simulink model "gm_uz_pmsm_model_6LUT_pd_vnl"  (R2023b)
settings: Solver=FixedStepAuto  StartTime=0.0  StopTime=0.05  RelTol=1e-3
PreLoadFcn:
  | uz_pmsm_model_init_parameter
PostLoadFcn:
  | % Import the data from Excel for a lookup table
  | FluxMapData = readtable('C:\Users\Philipp\ultrazohm\ultrazohm_sw\ip_cores\uz_pmsm_model\FluxMapData_2023-05-26_13-07-57.csv');
  | % Row indices for lookup table
  | d_current_in_d_axis = FluxMapData(8:27,1:end);
  | % Column indices for lookup table
  | q_current_in_d_axis = FluxMapData(29:48,1:end);
  | % Output values for lookup table
  | d_Flux_d_axis = FluxMapData(50:69,1:end);
undefined symbols (not defined in the file or in its folder): ad1, ad2, ad3, ad4, ad5, ad6, aq1, aq2, aq3, aq4, aq5, aq6, d_current_d_Flux, d_current_q_Flux, entkopplung_dynamic, entkopplung_linear, entkopplung_static, Fid1_Giq1, Fid2_Giq2, Flux_d, Flux_q, friction_coefficient, inertia, Ki_Bo_d, Ki_Bo_q, Kp_Bo_d, Kp_Bo_q, L_d, L_q, Ldq, parameter_nachfuerung, polepair, praediktion_entkopplung_nonlinear, psi_pm, q_current_d_Flux, q_current_q_Flux, R_1, simulate_mechanical, simulate_nonlinear_modell, simulate_open_loop, static_friction_torque, tau_sum, ts, ts_regler
libraries: hdlmdlgenlib x19, simulink x2, slpidlib x2
(part 3 of 4)

== system gm_uz_pmsm_model_6LUT_pd_vnl/Current_Controller/Psi_d_q ==
  I_d_set : Inport
  I_d : Inport  Port=2
  I_q_set : Inport  Port=3
  I_q : Inport  Port=4
  Flux_d Lookup Table : Lookup_n-D  BreakpointsForDimension1=d_current_d_Flux  BreakpointsForDimension2=q_current_d_Flux  BreakpointsForDimension3=[5, 7]  Table=Flux_d  InternalRulePriority=Speed  RndMeth=Simplest
      settings: InputPortMap=u0,u1
  Flux_d Lookup Table1 : Lookup_n-D  BreakpointsForDimension1=d_current_d_Flux  BreakpointsForDimension2=q_current_d_Flux  BreakpointsForDimension3=[5, 7]  Table=Flux_d  InternalRulePriority=Speed  RndMeth=Simplest
      settings: InputPortMap=u0,u1
  Flux_q Lookup Table1 : Lookup_n-D  BreakpointsForDimension1=d_current_q_Flux  BreakpointsForDimension2=q_current_q_Flux  BreakpointsForDimension3=[5, 7]  Table=Flux_q  InternalRulePriority=Speed  RndMeth=Simplest
      settings: InputPortMap=u0,u1
  Flux_q Lookup Table2 : Lookup_n-D  BreakpointsForDimension1=d_current_q_Flux  BreakpointsForDimension2=q_current_q_Flux  BreakpointsForDimension3=[5, 7]  Table=Flux_q  InternalRulePriority=Speed  RndMeth=Simplest
      settings: InputPortMap=u0,u1
  Ldq Lookup Table : Lookup_n-D  BreakpointsForDimension1=d_current_q_Flux  BreakpointsForDimension2=q_current_q_Flux  BreakpointsForDimension3=[5, 7]  Table=Ldq  ExtrapMethod=Clip  UseLastTableValue=on  InternalRulePriority=Speed  OutDataTypeStr=Inherit: Inherit from 'Table data'  RndMeth=Simplest
      settings: InputPortMap=u0,u1
  Lqd Lookup Table1 : Lookup_n-D  BreakpointsForDimension1=d_current_q_Flux  BreakpointsForDimension2=q_current_q_Flux  BreakpointsForDimension3=[5, 7]  Table=Ldq  ExtrapMethod=Clip  UseLastTableValue=on  InternalRulePriority=Speed  OutDataTypeStr=Inherit: Inherit from 'Table data'  RndMeth=Simplest
      settings: InputPortMap=u0,u1
  Scope : Scope  NumInputPorts=4
  psi_d_set : Outport
  psi_q_set : Outport  Port=2
  psi_d_LUT : Outport  Port=3
  psi_q_LUT : Outport  Port=4
  Ldq_LUT : Outport  Port=5
  Lqd_LUT : Outport  Port=6
  wires:
  I_d_set/1 -> Scope/1, Flux_d Lookup Table1/1
  I_q_set/1 -> Scope/2, Flux_q Lookup Table2/2
  Flux_d Lookup Table1/1 -> psi_d_set/1  "psi_d_set"
  Flux_q Lookup Table2/1 -> psi_q_set/1  "psi_q_set"
  Flux_d Lookup Table/1 -> psi_d_LUT/1  "psi_d_controller"
  Flux_q Lookup Table1/1 -> psi_q_LUT/1  "psi_q_controller"
  Ldq Lookup Table/1 -> Ldq_LUT/1  "Ldq_Karte"
  Lqd Lookup Table1/1 -> Lqd_LUT/1  "Ldq_Karte"
  I_d/1 -> Scope/3, Flux_q Lookup Table2/1, Lqd Lookup Table1/1, Ldq Lookup Table/1, Flux_q Lookup Table1/1, Flux_d Lookup Table/1
  I_q/1 -> Scope/4, Lqd Lookup Table1/2, Ldq Lookup Table/2, Flux_q Lookup Table1/2, Flux_d Lookup Table1/2, Flux_d Lookup Table/2

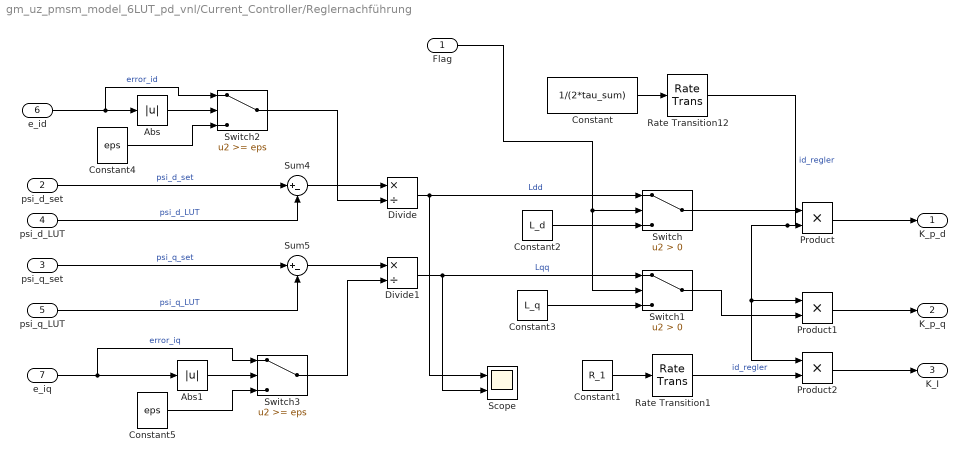
== system gm_uz_pmsm_model_6LUT_pd_vnl/Current_Controller/Reglernachführung ==
  Flag : Inport
  psi_d_set : Inport  Port=2
  psi_q_set : Inport  Port=3
  psi_d_LUT : Inport  Port=4
  psi_q_LUT : Inport  Port=5
  e_id : Inport  Port=6
  e_iq : Inport  Port=7
  Abs : Abs  SaturateOnIntegerOverflow=off
  Abs1 : Abs  SaturateOnIntegerOverflow=off
  Constant : Constant  Value=1/(2*tau_sum)
  Constant1 : Constant  Value=R_1
  Constant2 : Constant  Value=L_d
  Constant3 : Constant  Value=L_q
  Constant4 : Constant  Value=eps  SampleTime=ts_regler
  Constant5 : Constant  Value=eps  SampleTime=ts_regler
  Divide : Product  Inputs=*/
  Divide1 : Product  Inputs=*/
  Product : Product
  Product1 : Product
  Product2 : Product
  Rate Transition1 : RateTransition  OutPortSampleTime=ts_regler
  Rate Transition12 : RateTransition  OutPortSampleTime=ts_regler
  Scope : Scope  NumInputPorts=2
  Sum4 : Sum  Inputs=|+-
  Sum5 : Sum  Inputs=|+-
  Switch : Switch  Criteria=u2 > Threshold  SaturateOnIntegerOverflow=off  InputSameDT=off
  Switch1 : Switch  Criteria=u2 > Threshold  SaturateOnIntegerOverflow=off  InputSameDT=off
  Switch2 : Switch  Threshold=eps  SaturateOnIntegerOverflow=off  InputSameDT=off
  Switch3 : Switch  Threshold=eps  SaturateOnIntegerOverflow=off  InputSameDT=off
  K_p_d : Outport
  K_p_q : Outport  Port=2
  K_I : Outport  Port=3
  wires:
  Constant/1 -> Rate Transition12/1
  Product/1 -> K_p_d/1
  Product1/1 -> K_p_q/1
  Product2/1 -> K_I/1
  Constant1/1 -> Rate Transition1/1
  Rate Transition12/1 -> Product2/1, Product1/1, Product/2  "id_regler"
  Rate Transition1/1 -> Product2/2  "id_regler"
  Flag/1 -> Switch/2, Switch1/2
  Constant2/1 -> Switch/3
  Switch/1 -> Product/1
  Constant3/1 -> Switch1/3
  Switch1/1 -> Product1/2
  Sum4/1 -> Divide/1
  psi_q_LUT/1 -> Sum5/2  "psi_q_LUT"
  Sum5/1 -> Divide1/1
  psi_d_LUT/1 -> Sum4/2  "psi_d_LUT"
  psi_d_set/1 -> Sum4/1  "psi_d_set"
  psi_q_set/1 -> Sum5/1  "psi_q_set"
  Divide/1 -> Scope/1, Switch/1  "Ldd"
  Divide1/1 -> Scope/2, Switch1/1  "Lqq"
  e_id/1 -> Switch2/1, Abs/1  "error_id"
  Constant4/1 -> Switch2/3
  Abs/1 -> Switch2/2
  Switch2/1 -> Divide/2
  e_iq/1 -> Switch3/1, Abs1/1  "error_iq"
  Switch3/1 -> Divide1/2
  Abs1/1 -> Switch3/2
  Constant5/1 -> Switch3/3

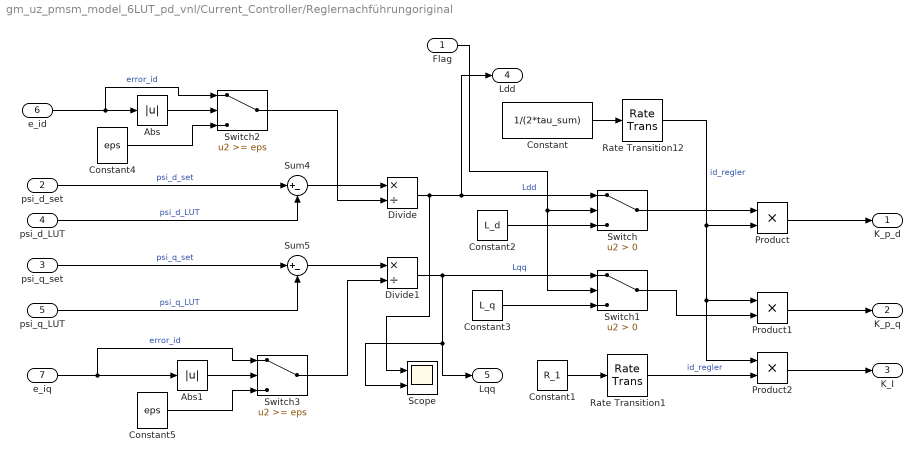
== system gm_uz_pmsm_model_6LUT_pd_vnl/Current_Controller/Reglernachführungoriginal ==
  Flag : Inport
  psi_d_set : Inport  Port=2
  psi_q_set : Inport  Port=3
  psi_d_LUT : Inport  Port=4
  psi_q_LUT : Inport  Port=5
  e_id : Inport  Port=6
  e_iq : Inport  Port=7
  Abs : Abs  SaturateOnIntegerOverflow=off
  Abs1 : Abs  SaturateOnIntegerOverflow=off
  Constant : Constant  Value=1/(2*tau_sum)
  Constant1 : Constant  Value=R_1
  Constant2 : Constant  Value=L_d
  Constant3 : Constant  Value=L_q
  Constant4 : Constant  Value=eps  SampleTime=ts_regler
  Constant5 : Constant  Value=eps  SampleTime=ts_regler
  Divide : Product  Inputs=*/
  Divide1 : Product  Inputs=*/
  Product : Product
  Product1 : Product
  Product2 : Product
  Rate Transition1 : RateTransition  OutPortSampleTime=ts_regler
  Rate Transition12 : RateTransition  OutPortSampleTime=ts_regler
  Scope : Scope  NumInputPorts=2
  Sum4 : Sum  Inputs=|+-
  Sum5 : Sum  Inputs=|+-
  Switch : Switch  Criteria=u2 > Threshold  SaturateOnIntegerOverflow=off  InputSameDT=off
  Switch1 : Switch  Criteria=u2 > Threshold  SaturateOnIntegerOverflow=off  InputSameDT=off
  Switch2 : Switch  Threshold=eps  SaturateOnIntegerOverflow=off  InputSameDT=off
  Switch3 : Switch  Threshold=eps  SaturateOnIntegerOverflow=off  InputSameDT=off
  K_p_d : Outport
  K_p_q : Outport  Port=2
  K_I : Outport  Port=3
  Ldd : Outport  Port=4
  Lqq : Outport  Port=5
  wires:
  Constant/1 -> Rate Transition12/1
  Product/1 -> K_p_d/1
  Product1/1 -> K_p_q/1
  Product2/1 -> K_I/1
  Constant1/1 -> Rate Transition1/1
  Rate Transition12/1 -> Product2/1, Product1/1, Product/2  "id_regler"
  Rate Transition1/1 -> Product2/2  "id_regler"
  Flag/1 -> Switch/2, Switch1/2
  Constant2/1 -> Switch/3
  Switch/1 -> Product/1
  Constant3/1 -> Switch1/3
  Switch1/1 -> Product1/2
  Sum4/1 -> Divide/1
  psi_q_LUT/1 -> Sum5/2  "psi_q_LUT"
  Sum5/1 -> Divide1/1
  psi_d_LUT/1 -> Sum4/2  "psi_d_LUT"
  psi_d_set/1 -> Sum4/1  "psi_d_set"
  psi_q_set/1 -> Sum5/1  "psi_q_set"
  Divide/1 -> Scope/1, Ldd/1, Switch/1  "Ldd"
  Divide1/1 -> Scope/2, Lqq/1, Switch1/1  "Lqq"
  e_id/1 -> Switch2/1, Abs/1  "error_id"
  Constant4/1 -> Switch2/3
  Abs/1 -> Switch2/2
  Switch2/1 -> Divide/2
  e_iq/1 -> Switch3/1, Abs1/1  "error_id"
  Switch3/1 -> Divide1/2
  Abs1/1 -> Switch3/2
  Constant5/1 -> Switch3/3

== system gm_uz_pmsm_model_6LUT_pd_vnl/uz_pmsm_model_6LUT/Abs ==
  In1 : Inport
  Abs : Abs  SampleTime=1e-08  OutDataTypeStr=double  SaturateOnIntegerOverflow=off
  Out1 : Outport
  wires:
  Abs/1 -> Out1/1
  In1/1 -> Abs/1

== system gm_uz_pmsm_model_6LUT_pd_vnl/uz_pmsm_model_6LUT/Data Type Conversion1 ==
  In1 : Inport
  Data Type Conversion1 : DataTypeConversion  OutDataTypeStr=double  RndMeth=Nearest  SampleTime=1e-08  SaturateOnIntegerOverflow=off
  Data Type Conversion1_pd1 : Delay  DelayLength=3
  Out1 : Outport
  wires:
  Data Type Conversion1_pd1/1 -> Out1/1
  Data Type Conversion1/1 -> Data Type Conversion1_pd1/1
  In1/1 -> Data Type Conversion1/1

== system gm_uz_pmsm_model_6LUT_pd_vnl/uz_pmsm_model_6LUT/Data Type Conversion10 ==
  In1 : Inport
  Data Type Conversion10 : DataTypeConversion  OutDataTypeStr=double  RndMeth=Nearest  SampleTime=1e-08  SaturateOnIntegerOverflow=off
  Data Type Conversion10_pd1 : Delay  DelayLength=3
  Out1 : Outport
  wires:
  Data Type Conversion10_pd1/1 -> Out1/1
  Data Type Conversion10/1 -> Data Type Conversion10_pd1/1
  In1/1 -> Data Type Conversion10/1

== system gm_uz_pmsm_model_6LUT_pd_vnl/uz_pmsm_model_6LUT/Data Type Conversion11 ==
  In1 : Inport
  Data Type Conversion11 : DataTypeConversion  OutDataTypeStr=double  RndMeth=Nearest  SampleTime=1e-08  SaturateOnIntegerOverflow=off
  Data Type Conversion11_pd1 : Delay  DelayLength=3
  Out1 : Outport
  wires:
  Data Type Conversion11_pd1/1 -> Out1/1
  Data Type Conversion11/1 -> Data Type Conversion11_pd1/1
  In1/1 -> Data Type Conversion11/1

== system gm_uz_pmsm_model_6LUT_pd_vnl/uz_pmsm_model_6LUT/Data Type Conversion111 ==
  In1 : Inport
  Data Type Conversion111 : DataTypeConversion  OutDataTypeStr=single  RndMeth=Nearest  SampleTime=1e-08  SaturateOnIntegerOverflow=off
  Data Type Conversion111_pd1 : Delay  DelayLength=3
  Out1 : Outport
  wires:
  Data Type Conversion111_pd1/1 -> Out1/1
  Data Type Conversion111/1 -> Data Type Conversion111_pd1/1
  In1/1 -> Data Type Conversion111/1

== system gm_uz_pmsm_model_6LUT_pd_vnl/uz_pmsm_model_6LUT/Data Type Conversion12 ==
  In1 : Inport
  Data Type Conversion12 : DataTypeConversion  OutDataTypeStr=double  RndMeth=Nearest  SampleTime=1e-08  SaturateOnIntegerOverflow=off
  Data Type Conversion12_pd1 : Delay  DelayLength=3
  Out1 : Outport
  wires:
  Data Type Conversion12_pd1/1 -> Out1/1
  Data Type Conversion12/1 -> Data Type Conversion12_pd1/1
  In1/1 -> Data Type Conversion12/1

== system gm_uz_pmsm_model_6LUT_pd_vnl/uz_pmsm_model_6LUT/Data Type Conversion121 ==
  In1 : Inport
  Data Type Conversion121 : DataTypeConversion  OutDataTypeStr=double  RndMeth=Nearest  SampleTime=1e-08  SaturateOnIntegerOverflow=off
  Data Type Conversion121_pd1 : Delay  DelayLength=3
  Out1 : Outport
  wires:
  Data Type Conversion121_pd1/1 -> Out1/1
  Data Type Conversion121/1 -> Data Type Conversion121_pd1/1
  In1/1 -> Data Type Conversion121/1

== system gm_uz_pmsm_model_6LUT_pd_vnl/uz_pmsm_model_6LUT/Data Type Conversion13 ==
  In1 : Inport
  Data Type Conversion13 : DataTypeConversion  OutDataTypeStr=double  RndMeth=Nearest  SampleTime=1e-08  SaturateOnIntegerOverflow=off
  Data Type Conversion13_pd1 : Delay  DelayLength=3
  Out1 : Outport
  wires:
  Data Type Conversion13_pd1/1 -> Out1/1
  Data Type Conversion13/1 -> Data Type Conversion13_pd1/1
  In1/1 -> Data Type Conversion13/1

== system gm_uz_pmsm_model_6LUT_pd_vnl/uz_pmsm_model_6LUT/Data Type Conversion14 ==
  In1 : Inport
  Data Type Conversion14 : DataTypeConversion  OutDataTypeStr=double  RndMeth=Nearest  SampleTime=1e-08  SaturateOnIntegerOverflow=off
  Data Type Conversion14_pd1 : Delay  DelayLength=3
  Out1 : Outport
  wires:
  Data Type Conversion14_pd1/1 -> Out1/1
  Data Type Conversion14/1 -> Data Type Conversion14_pd1/1
  In1/1 -> Data Type Conversion14/1

== system gm_uz_pmsm_model_6LUT_pd_vnl/uz_pmsm_model_6LUT/Data Type Conversion15 ==
  In1 : Inport
  Data Type Conversion15 : DataTypeConversion  OutDataTypeStr=single  RndMeth=Nearest  SampleTime=1e-08  SaturateOnIntegerOverflow=off
  Data Type Conversion15_pd1 : Delay  DelayLength=3
  Out1 : Outport
  wires:
  Data Type Conversion15_pd1/1 -> Out1/1
  Data Type Conversion15/1 -> Data Type Conversion15_pd1/1
  In1/1 -> Data Type Conversion15/1

== system gm_uz_pmsm_model_6LUT_pd_vnl/uz_pmsm_model_6LUT/Data Type Conversion16 ==
  In1 : Inport
  Data Type Conversion16 : DataTypeConversion  OutDataTypeStr=single  RndMeth=Nearest  SampleTime=1e-08  SaturateOnIntegerOverflow=off
  Data Type Conversion16_pd1 : Delay  DelayLength=3
  Out1 : Outport
  wires:
  Data Type Conversion16_pd1/1 -> Out1/1
  Data Type Conversion16/1 -> Data Type Conversion16_pd1/1
  In1/1 -> Data Type Conversion16/1

== system gm_uz_pmsm_model_6LUT_pd_vnl/uz_pmsm_model_6LUT/Data Type Conversion17 ==
  In1 : Inport
  Data Type Conversion17 : DataTypeConversion  OutDataTypeStr=single  RndMeth=Nearest  SampleTime=1e-08  SaturateOnIntegerOverflow=off
  Data Type Conversion17_pd1 : Delay  DelayLength=3
  Out1 : Outport
  wires:
  Data Type Conversion17_pd1/1 -> Out1/1
  Data Type Conversion17/1 -> Data Type Conversion17_pd1/1
  In1/1 -> Data Type Conversion17/1

== system gm_uz_pmsm_model_6LUT_pd_vnl/uz_pmsm_model_6LUT/Data Type Conversion2 ==
  In1 : Inport
  Data Type Conversion2 : DataTypeConversion  OutDataTypeStr=double  RndMeth=Nearest  SampleTime=1e-08  SaturateOnIntegerOverflow=off
  Data Type Conversion2_pd1 : Delay  DelayLength=3
  Out1 : Outport
  wires:
  Data Type Conversion2_pd1/1 -> Out1/1
  Data Type Conversion2/1 -> Data Type Conversion2_pd1/1
  In1/1 -> Data Type Conversion2/1

== system gm_uz_pmsm_model_6LUT_pd_vnl/uz_pmsm_model_6LUT/Data Type Conversion21 ==
  In1 : Inport
  Data Type Conversion21 : DataTypeConversion  OutDataTypeStr=double  RndMeth=Nearest  SampleTime=1e-08  SaturateOnIntegerOverflow=off
  Data Type Conversion21_pd1 : Delay  DelayLength=3
  Out1 : Outport
  wires:
  Data Type Conversion21_pd1/1 -> Out1/1
  Data Type Conversion21/1 -> Data Type Conversion21_pd1/1
  In1/1 -> Data Type Conversion21/1

== system gm_uz_pmsm_model_6LUT_pd_vnl/uz_pmsm_model_6LUT/Data Type Conversion22 ==
  In1 : Inport
  Data Type Conversion22 : DataTypeConversion  OutDataTypeStr=double  RndMeth=Nearest  SampleTime=1e-08  SaturateOnIntegerOverflow=off
  Data Type Conversion22_pd1 : Delay  DelayLength=3
  Out1 : Outport
  wires:
  Data Type Conversion22_pd1/1 -> Out1/1
  Data Type Conversion22/1 -> Data Type Conversion22_pd1/1
  In1/1 -> Data Type Conversion22/1

== system gm_uz_pmsm_model_6LUT_pd_vnl/uz_pmsm_model_6LUT/Data Type Conversion23 ==
  In1 : Inport
  Data Type Conversion23 : DataTypeConversion  OutDataTypeStr=double  RndMeth=Nearest  SampleTime=1e-08  SaturateOnIntegerOverflow=off
  Data Type Conversion23_pd1 : Delay  DelayLength=3
  Out1 : Outport
  wires:
  Data Type Conversion23_pd1/1 -> Out1/1
  Data Type Conversion23/1 -> Data Type Conversion23_pd1/1
  In1/1 -> Data Type Conversion23/1

== system gm_uz_pmsm_model_6LUT_pd_vnl/uz_pmsm_model_6LUT/Data Type Conversion24 ==
  In1 : Inport
  Data Type Conversion24 : DataTypeConversion  OutDataTypeStr=double  RndMeth=Nearest  SampleTime=1e-08  SaturateOnIntegerOverflow=off
  Data Type Conversion24_pd1 : Delay  DelayLength=3
  Out1 : Outport
  wires:
  Data Type Conversion24_pd1/1 -> Out1/1
  Data Type Conversion24/1 -> Data Type Conversion24_pd1/1
  In1/1 -> Data Type Conversion24/1

== system gm_uz_pmsm_model_6LUT_pd_vnl/uz_pmsm_model_6LUT/Data Type Conversion3 ==
  In1 : Inport
  Data Type Conversion3 : DataTypeConversion  OutDataTypeStr=double  RndMeth=Nearest  SampleTime=1e-08  SaturateOnIntegerOverflow=off
  Data Type Conversion3_pd1 : Delay  DelayLength=3
  Out1 : Outport
  wires:
  Data Type Conversion3_pd1/1 -> Out1/1
  Data Type Conversion3/1 -> Data Type Conversion3_pd1/1
  In1/1 -> Data Type Conversion3/1

== system gm_uz_pmsm_model_6LUT_pd_vnl/uz_pmsm_model_6LUT/Data Type Conversion31 ==
  In1 : Inport
  Data Type Conversion31 : DataTypeConversion  OutDataTypeStr=double  RndMeth=Nearest  SampleTime=1e-08  SaturateOnIntegerOverflow=off
  Data Type Conversion31_pd1 : Delay  DelayLength=3
  Out1 : Outport
  wires:
  Data Type Conversion31_pd1/1 -> Out1/1
  Data Type Conversion31/1 -> Data Type Conversion31_pd1/1
  In1/1 -> Data Type Conversion31/1

== system gm_uz_pmsm_model_6LUT_pd_vnl/uz_pmsm_model_6LUT/Data Type Conversion32 ==
  In1 : Inport
  Data Type Conversion32 : DataTypeConversion  OutDataTypeStr=double  RndMeth=Nearest  SampleTime=1e-08  SaturateOnIntegerOverflow=off
  Data Type Conversion32_pd1 : Delay  DelayLength=3
  Out1 : Outport
  wires:
  Data Type Conversion32_pd1/1 -> Out1/1
  Data Type Conversion32/1 -> Data Type Conversion32_pd1/1
  In1/1 -> Data Type Conversion32/1

== system gm_uz_pmsm_model_6LUT_pd_vnl/uz_pmsm_model_6LUT/Data Type Conversion4 ==
  In1 : Inport
  Data Type Conversion4 : DataTypeConversion  OutDataTypeStr=double  RndMeth=Nearest  SampleTime=1e-08  SaturateOnIntegerOverflow=off
  Data Type Conversion4_pd1 : Delay  DelayLength=3
  Out1 : Outport
  wires:
  Data Type Conversion4_pd1/1 -> Out1/1
  Data Type Conversion4/1 -> Data Type Conversion4_pd1/1
  In1/1 -> Data Type Conversion4/1

== system gm_uz_pmsm_model_6LUT_pd_vnl/uz_pmsm_model_6LUT/Data Type Conversion41 ==
  In1 : Inport
  Data Type Conversion41 : DataTypeConversion  OutDataTypeStr=single  RndMeth=Nearest  SampleTime=1e-08  SaturateOnIntegerOverflow=off
  Data Type Conversion41_pd1 : Delay  DelayLength=3
  Out1 : Outport
  wires:
  Data Type Conversion41_pd1/1 -> Out1/1
  Data Type Conversion41/1 -> Data Type Conversion41_pd1/1
  In1/1 -> Data Type Conversion41/1

== system gm_uz_pmsm_model_6LUT_pd_vnl/uz_pmsm_model_6LUT/Data Type Conversion42 ==
  In1 : Inport
  Data Type Conversion42 : DataTypeConversion  OutDataTypeStr=double  RndMeth=Nearest  SampleTime=1e-08  SaturateOnIntegerOverflow=off
  Data Type Conversion42_pd1 : Delay  DelayLength=3
  Out1 : Outport
  wires:
  Data Type Conversion42_pd1/1 -> Out1/1
  Data Type Conversion42/1 -> Data Type Conversion42_pd1/1
  In1/1 -> Data Type Conversion42/1

== system gm_uz_pmsm_model_6LUT_pd_vnl/uz_pmsm_model_6LUT/Data Type Conversion43 ==
  In1 : Inport
  Data Type Conversion43 : DataTypeConversion  OutDataTypeStr=double  RndMeth=Nearest  SampleTime=1e-08  SaturateOnIntegerOverflow=off
  Data Type Conversion43_pd1 : Delay  DelayLength=3
  Out1 : Outport
  wires:
  Data Type Conversion43_pd1/1 -> Out1/1
  Data Type Conversion43/1 -> Data Type Conversion43_pd1/1
  In1/1 -> Data Type Conversion43/1

== system gm_uz_pmsm_model_6LUT_pd_vnl/uz_pmsm_model_6LUT/Data Type Conversion5 ==
  In1 : Inport
  Data Type Conversion5 : DataTypeConversion  OutDataTypeStr=double  RndMeth=Nearest  SampleTime=1e-08  SaturateOnIntegerOverflow=off
  Data Type Conversion5_pd1 : Delay  DelayLength=3
  Out1 : Outport
  wires:
  Data Type Conversion5_pd1/1 -> Out1/1
  Data Type Conversion5/1 -> Data Type Conversion5_pd1/1
  In1/1 -> Data Type Conversion5/1

== system gm_uz_pmsm_model_6LUT_pd_vnl/uz_pmsm_model_6LUT/Data Type Conversion51 ==
  In1 : Inport
  Data Type Conversion51 : DataTypeConversion  OutDataTypeStr=single  RndMeth=Nearest  SampleTime=1e-08  SaturateOnIntegerOverflow=off
  Data Type Conversion51_pd1 : Delay  DelayLength=3
  Out1 : Outport
  wires:
  Data Type Conversion51_pd1/1 -> Out1/1
  Data Type Conversion51/1 -> Data Type Conversion51_pd1/1
  In1/1 -> Data Type Conversion51/1

== system gm_uz_pmsm_model_6LUT_pd_vnl/uz_pmsm_model_6LUT/Data Type Conversion52 ==
  In1 : Inport
  Data Type Conversion52 : DataTypeConversion  OutDataTypeStr=single  RndMeth=Nearest  SampleTime=1e-08  SaturateOnIntegerOverflow=off
  Data Type Conversion52_pd1 : Delay  DelayLength=3
  Out1 : Outport
  wires:
  Data Type Conversion52_pd1/1 -> Out1/1
  Data Type Conversion52/1 -> Data Type Conversion52_pd1/1
  In1/1 -> Data Type Conversion52/1

== system gm_uz_pmsm_model_6LUT_pd_vnl/uz_pmsm_model_6LUT/Data Type Conversion53 ==
  In1 : Inport
  Data Type Conversion53 : DataTypeConversion  OutDataTypeStr=single  RndMeth=Nearest  SampleTime=1e-08  SaturateOnIntegerOverflow=off
  Data Type Conversion53_pd1 : Delay  DelayLength=3
  Out1 : Outport
  wires:
  Data Type Conversion53_pd1/1 -> Out1/1
  Data Type Conversion53/1 -> Data Type Conversion53_pd1/1
  In1/1 -> Data Type Conversion53/1

== system gm_uz_pmsm_model_6LUT_pd_vnl/uz_pmsm_model_6LUT/Data Type Conversion6 ==
  In1 : Inport
  Data Type Conversion6 : DataTypeConversion  OutDataTypeStr=single  RndMeth=Nearest  SampleTime=1e-08  SaturateOnIntegerOverflow=off
  Data Type Conversion6_pd1 : Delay  DelayLength=3
  Out1 : Outport
  wires:
  Data Type Conversion6_pd1/1 -> Out1/1
  Data Type Conversion6/1 -> Data Type Conversion6_pd1/1
  In1/1 -> Data Type Conversion6/1

== system gm_uz_pmsm_model_6LUT_pd_vnl/uz_pmsm_model_6LUT/Data Type Conversion61 ==
  In1 : Inport
  Data Type Conversion61 : DataTypeConversion  OutDataTypeStr=single  RndMeth=Nearest  SampleTime=1e-08  SaturateOnIntegerOverflow=off
  Data Type Conversion61_pd1 : Delay  DelayLength=3
  Out1 : Outport
  wires:
  Data Type Conversion61_pd1/1 -> Out1/1
  Data Type Conversion61/1 -> Data Type Conversion61_pd1/1
  In1/1 -> Data Type Conversion61/1

== system gm_uz_pmsm_model_6LUT_pd_vnl/uz_pmsm_model_6LUT/Data Type Conversion62 ==
  In1 : Inport
  Data Type Conversion62 : DataTypeConversion  OutDataTypeStr=double  RndMeth=Nearest  SampleTime=1e-08  SaturateOnIntegerOverflow=off
  Data Type Conversion62_pd1 : Delay  DelayLength=3
  Out1 : Outport
  wires:
  Data Type Conversion62_pd1/1 -> Out1/1
  Data Type Conversion62/1 -> Data Type Conversion62_pd1/1
  In1/1 -> Data Type Conversion62/1

== system gm_uz_pmsm_model_6LUT_pd_vnl/uz_pmsm_model_6LUT/Data Type Conversion63 ==
  In1 : Inport
  Data Type Conversion63 : DataTypeConversion  OutDataTypeStr=single  RndMeth=Nearest  SampleTime=1e-08  SaturateOnIntegerOverflow=off
  Data Type Conversion63_pd1 : Delay  DelayLength=3
  Out1 : Outport
  wires:
  Data Type Conversion63_pd1/1 -> Out1/1
  Data Type Conversion63/1 -> Data Type Conversion63_pd1/1
  In1/1 -> Data Type Conversion63/1

== system gm_uz_pmsm_model_6LUT_pd_vnl/uz_pmsm_model_6LUT/Data Type Conversion64 ==
  In1 : Inport
  Data Type Conversion64 : DataTypeConversion  OutDataTypeStr=double  RndMeth=Nearest  SampleTime=1e-08  SaturateOnIntegerOverflow=off
  Data Type Conversion64_pd1 : Delay  DelayLength=3
  Out1 : Outport
  wires:
  Data Type Conversion64_pd1/1 -> Out1/1
  Data Type Conversion64/1 -> Data Type Conversion64_pd1/1
  In1/1 -> Data Type Conversion64/1

== system gm_uz_pmsm_model_6LUT_pd_vnl/uz_pmsm_model_6LUT/Data Type Conversion7 ==
  In1 : Inport
  Data Type Conversion7 : DataTypeConversion  OutDataTypeStr=single  RndMeth=Nearest  SampleTime=1e-08  SaturateOnIntegerOverflow=off
  Data Type Conversion7_pd1 : Delay  DelayLength=3
  Out1 : Outport
  wires:
  Data Type Conversion7_pd1/1 -> Out1/1
  Data Type Conversion7/1 -> Data Type Conversion7_pd1/1
  In1/1 -> Data Type Conversion7/1

== system gm_uz_pmsm_model_6LUT_pd_vnl/uz_pmsm_model_6LUT/Data Type Conversion71 ==
  In1 : Inport
  Data Type Conversion71 : DataTypeConversion  OutDataTypeStr=single  RndMeth=Nearest  SampleTime=1e-08  SaturateOnIntegerOverflow=off
  Data Type Conversion71_pd1 : Delay  DelayLength=3
  Out1 : Outport
  wires:
  Data Type Conversion71_pd1/1 -> Out1/1
  Data Type Conversion71/1 -> Data Type Conversion71_pd1/1
  In1/1 -> Data Type Conversion71/1

== system gm_uz_pmsm_model_6LUT_pd_vnl/uz_pmsm_model_6LUT/Data Type Conversion72 ==
  In1 : Inport
  Data Type Conversion72 : DataTypeConversion  OutDataTypeStr=double  RndMeth=Nearest  SampleTime=1e-08  SaturateOnIntegerOverflow=off
  Data Type Conversion72_pd1 : Delay  DelayLength=3
  Out1 : Outport
  wires:
  Data Type Conversion72_pd1/1 -> Out1/1
  Data Type Conversion72/1 -> Data Type Conversion72_pd1/1
  In1/1 -> Data Type Conversion72/1

== system gm_uz_pmsm_model_6LUT_pd_vnl/uz_pmsm_model_6LUT/Data Type Conversion8 ==
  In1 : Inport
  Data Type Conversion8 : DataTypeConversion  OutDataTypeStr=double  RndMeth=Nearest  SampleTime=1e-08  SaturateOnIntegerOverflow=off
  Data Type Conversion8_pd1 : Delay  DelayLength=3
  Out1 : Outport
  wires:
  Data Type Conversion8_pd1/1 -> Out1/1
  Data Type Conversion8/1 -> Data Type Conversion8_pd1/1
  In1/1 -> Data Type Conversion8/1

== system gm_uz_pmsm_model_6LUT_pd_vnl/uz_pmsm_model_6LUT/Data Type Conversion81 ==
  In1 : Inport
  Data Type Conversion81 : DataTypeConversion  OutDataTypeStr=single  RndMeth=Nearest  SampleTime=1e-08  SaturateOnIntegerOverflow=off
  Data Type Conversion81_pd1 : Delay  DelayLength=3
  Out1 : Outport
  wires:
  Data Type Conversion81_pd1/1 -> Out1/1
  Data Type Conversion81/1 -> Data Type Conversion81_pd1/1
  In1/1 -> Data Type Conversion81/1

== system gm_uz_pmsm_model_6LUT_pd_vnl/uz_pmsm_model_6LUT/Data Type Conversion82 ==
  In1 : Inport
  Data Type Conversion82 : DataTypeConversion  OutDataTypeStr=single  RndMeth=Nearest  SampleTime=1e-08  SaturateOnIntegerOverflow=off
  Data Type Conversion82_pd1 : Delay  DelayLength=3
  Out1 : Outport
  wires:
  Data Type Conversion82_pd1/1 -> Out1/1
  Data Type Conversion82/1 -> Data Type Conversion82_pd1/1
  In1/1 -> Data Type Conversion82/1

== system gm_uz_pmsm_model_6LUT_pd_vnl/uz_pmsm_model_6LUT/Data Type Conversion83 ==
  In1 : Inport
  Data Type Conversion83 : DataTypeConversion  OutDataTypeStr=single  RndMeth=Nearest  SampleTime=1e-08  SaturateOnIntegerOverflow=off
  Data Type Conversion83_pd1 : Delay  DelayLength=3
  Out1 : Outport
  wires:
  Data Type Conversion83_pd1/1 -> Out1/1
  Data Type Conversion83/1 -> Data Type Conversion83_pd1/1
  In1/1 -> Data Type Conversion83/1

== system gm_uz_pmsm_model_6LUT_pd_vnl/uz_pmsm_model_6LUT/Data Type Conversion9 ==
  In1 : Inport
  Data Type Conversion9 : DataTypeConversion  OutDataTypeStr=double  RndMeth=Nearest  SampleTime=1e-08  SaturateOnIntegerOverflow=off
  Data Type Conversion9_pd1 : Delay  DelayLength=3
  Out1 : Outport
  wires:
  Data Type Conversion9_pd1/1 -> Out1/1
  Data Type Conversion9/1 -> Data Type Conversion9_pd1/1
  In1/1 -> Data Type Conversion9/1

== system gm_uz_pmsm_model_6LUT_pd_vnl/uz_pmsm_model_6LUT/Divide ==
  In1 : Inport
  In2 : Inport  Port=2
  Divide : Product  Inputs=**  OutDataTypeStr=double  SampleTime=1e-08
  Divide_pd1 : Delay  DelayLength=6
  Out1 : Outport
  wires:
  Divide_pd1/1 -> Out1/1
  Divide/1 -> Divide_pd1/1
  In2/1 -> Divide/2
  In1/1 -> Divide/1

== system gm_uz_pmsm_model_6LUT_pd_vnl/uz_pmsm_model_6LUT/Divide1 ==
  In1 : Inport
  In2 : Inport  Port=2
  Divide1 : Product  Inputs=*/  OutDataTypeStr=double  SampleTime=1e-08
  Divide1_pd1 : Delay  DelayLength=31
  Out1 : Outport
  wires:
  Divide1_pd1/1 -> Out1/1
  Divide1/1 -> Divide1_pd1/1
  In2/1 -> Divide1/2
  In1/1 -> Divide1/1

== system gm_uz_pmsm_model_6LUT_pd_vnl/uz_pmsm_model_6LUT/Divide_recip ==
  In1 : Inport
  Divide_recip : Math  Operator=reciprocal  SampleTime=1e-08
  Divide_recip_pd1 : Delay  DelayLength=30
  Out1 : Outport
  wires:
  Divide_recip_pd1/1 -> Out1/1
  Divide_recip/1 -> Divide_recip_pd1/1
  In1/1 -> Divide_recip/1

== system gm_uz_pmsm_model_6LUT_pd_vnl/uz_pmsm_model_6LUT/Factor ==
  In1 : Inport
  In2 : Inport  Port=2
  Factor : Product  Inputs=**  OutDataTypeStr=double  SampleTime=1e-08
  Factor_pd1 : Delay  DelayLength=6
  Out1 : Outport
  wires:
  Factor_pd1/1 -> Out1/1
  Factor/1 -> Factor_pd1/1
  In2/1 -> Factor/2
  In1/1 -> Factor/1

== system gm_uz_pmsm_model_6LUT_pd_vnl/uz_pmsm_model_6LUT/Gain ==
  In1 : Inport
  In2 : Inport  Port=2
  Gain : Product  Inputs=**  OutDataTypeStr=double  SampleTime=1e-08
  Gain_pd1 : Delay  DelayLength=6
  Out1 : Outport
  wires:
  Gain_pd1/1 -> Out1/1
  Gain/1 -> Gain_pd1/1
  In2/1 -> Gain/2
  In1/1 -> Gain/1

== system gm_uz_pmsm_model_6LUT_pd_vnl/uz_pmsm_model_6LUT/Gain7 ==
  In1 : Inport
  In2 : Inport  Port=2
  Gain7 : Product  Inputs=**  OutDataTypeStr=double  SampleTime=1e-08
  Gain7_pd1 : Delay  DelayLength=6
  Out1 : Outport
  wires:
  Gain7_pd1/1 -> Out1/1
  Gain7/1 -> Gain7_pd1/1
  In2/1 -> Gain7/2
  In1/1 -> Gain7/1

== system gm_uz_pmsm_model_6LUT_pd_vnl/uz_pmsm_model_6LUT/Gain71 ==
  In1 : Inport
  In2 : Inport  Port=2
  Gain71 : Product  Inputs=**  OutDataTypeStr=double  SampleTime=1e-08
  Gain71_pd1 : Delay  DelayLength=6
  Out1 : Outport
  wires:
  Gain71_pd1/1 -> Out1/1
  Gain71/1 -> Gain71_pd1/1
  In2/1 -> Gain71/2
  In1/1 -> Gain71/1

== system gm_uz_pmsm_model_6LUT_pd_vnl/uz_pmsm_model_6LUT/Gain_unaryminus ==
  In1 : Inport
  Gain_unaryminus : UnaryMinus  SampleTime=1e-08
  Out1 : Outport
  wires:
  Gain_unaryminus/1 -> Out1/1
  In1/1 -> Gain_unaryminus/1

== system gm_uz_pmsm_model_6LUT_pd_vnl/uz_pmsm_model_6LUT/Gain_unaryminus1 ==
  In1 : Inport
  Gain_unaryminus1 : UnaryMinus  SampleTime=1e-08
  Out1 : Outport
  wires:
  Gain_unaryminus1/1 -> Out1/1
  In1/1 -> Gain_unaryminus1/1

== system gm_uz_pmsm_model_6LUT_pd_vnl/uz_pmsm_model_6LUT/Log ==
  In1 : Inport
  Log : Math  Operator=log  SampleTime=1e-08
  Log_pd1 : Delay  DelayLength=20
  Out1 : Outport
  wires:
  Log_pd1/1 -> Out1/1
  Log/1 -> Log_pd1/1
  In1/1 -> Log/1

== system gm_uz_pmsm_model_6LUT_pd_vnl/uz_pmsm_model_6LUT/Log1 ==
  In1 : Inport
  Log1 : Math  Operator=log  SampleTime=1e-08
  Log1_pd1 : Delay  DelayLength=20
  Out1 : Outport
  wires:
  Log1_pd1/1 -> Out1/1
  Log1/1 -> Log1_pd1/1
  In1/1 -> Log1/1

== system gm_uz_pmsm_model_6LUT_pd_vnl/uz_pmsm_model_6LUT/Log11 ==
  In1 : Inport
  Log11 : Math  Operator=log  SampleTime=1e-08
  Log11_pd1 : Delay  DelayLength=20
  Out1 : Outport
  wires:
  Log11_pd1/1 -> Out1/1
  Log11/1 -> Log11_pd1/1
  In1/1 -> Log11/1

== system gm_uz_pmsm_model_6LUT_pd_vnl/uz_pmsm_model_6LUT/Log2 ==
  In1 : Inport
  Log2 : Math  Operator=log  SampleTime=1e-08
  Log2_pd1 : Delay  DelayLength=20
  Out1 : Outport
  wires:
  Log2_pd1/1 -> Out1/1
  Log2/1 -> Log2_pd1/1
  In1/1 -> Log2/1

== system gm_uz_pmsm_model_6LUT_pd_vnl/uz_pmsm_model_6LUT/Product ==
  In1 : Inport
  In2 : Inport  Port=2
  Product : Product  Inputs=**  OutDataTypeStr=double  SampleTime=1e-08
  Product_pd1 : Delay  DelayLength=6
  Out1 : Outport
  wires:
  Product_pd1/1 -> Out1/1
  Product/1 -> Product_pd1/1
  In2/1 -> Product/2
  In1/1 -> Product/1

== system gm_uz_pmsm_model_6LUT_pd_vnl/uz_pmsm_model_6LUT/Product1 ==
  In1 : Inport
  In2 : Inport  Port=2
  Product1 : Product  Inputs=**  OutDataTypeStr=double  SampleTime=1e-08
  Product1_pd1 : Delay  DelayLength=6
  Out1 : Outport
  wires:
  Product1_pd1/1 -> Out1/1
  Product1/1 -> Product1_pd1/1
  In2/1 -> Product1/2
  In1/1 -> Product1/1

== system gm_uz_pmsm_model_6LUT_pd_vnl/uz_pmsm_model_6LUT/Product10 ==
  In1 : Inport
  In2 : Inport  Port=2
  Product10 : Product  Inputs=**  OutDataTypeStr=double  SampleTime=1e-08
  Product10_pd1 : Delay  DelayLength=6
  Out1 : Outport
  wires:
  Product10_pd1/1 -> Out1/1
  Product10/1 -> Product10_pd1/1
  In2/1 -> Product10/2
  In1/1 -> Product10/1

== system gm_uz_pmsm_model_6LUT_pd_vnl/uz_pmsm_model_6LUT/Product101 ==
  In1 : Inport
  In2 : Inport  Port=2
  Product101 : Product  Inputs=**  OutDataTypeStr=double  SampleTime=1e-08
  Product101_pd1 : Delay  DelayLength=6
  Out1 : Outport
  wires:
  Product101_pd1/1 -> Out1/1
  Product101/1 -> Product101_pd1/1
  In2/1 -> Product101/2
  In1/1 -> Product101/1

== system gm_uz_pmsm_model_6LUT_pd_vnl/uz_pmsm_model_6LUT/Product102 ==
  In1 : Inport
  In2 : Inport  Port=2
  Product102 : Product  Inputs=**  OutDataTypeStr=double  SampleTime=1e-08
  Product102_pd1 : Delay  DelayLength=6
  Out1 : Outport
  wires:
  Product102_pd1/1 -> Out1/1
  Product102/1 -> Product102_pd1/1
  In2/1 -> Product102/2
  In1/1 -> Product102/1

== system gm_uz_pmsm_model_6LUT_pd_vnl/uz_pmsm_model_6LUT/Product103 ==
  In1 : Inport
  In2 : Inport  Port=2
  Product103 : Product  Inputs=**  OutDataTypeStr=double  SampleTime=1e-08
  Product103_pd1 : Delay  DelayLength=6
  Out1 : Outport
  wires:
  Product103_pd1/1 -> Out1/1
  Product103/1 -> Product103_pd1/1
  In2/1 -> Product103/2
  In1/1 -> Product103/1

== system gm_uz_pmsm_model_6LUT_pd_vnl/uz_pmsm_model_6LUT/Product104 ==
  In1 : Inport
  In2 : Inport  Port=2
  Product104 : Product  Inputs=**  OutDataTypeStr=double  SampleTime=1e-08
  Product104_pd1 : Delay  DelayLength=6
  Out1 : Outport
  wires:
  Product104_pd1/1 -> Out1/1
  Product104/1 -> Product104_pd1/1
  In2/1 -> Product104/2
  In1/1 -> Product104/1

== system gm_uz_pmsm_model_6LUT_pd_vnl/uz_pmsm_model_6LUT/Product105 ==
  In1 : Inport
  In2 : Inport  Port=2
  Product105 : Product  Inputs=**  OutDataTypeStr=double  SampleTime=1e-08
  Product105_pd1 : Delay  DelayLength=6
  Out1 : Outport
  wires:
  Product105_pd1/1 -> Out1/1
  Product105/1 -> Product105_pd1/1
  In2/1 -> Product105/2
  In1/1 -> Product105/1

== system gm_uz_pmsm_model_6LUT_pd_vnl/uz_pmsm_model_6LUT/Product11 ==
  In1 : Inport
  In2 : Inport  Port=2
  Product11 : Product  Inputs=**  OutDataTypeStr=double  SampleTime=1e-08
  Product11_pd1 : Delay  DelayLength=6
  Out1 : Outport
  wires:
  Product11_pd1/1 -> Out1/1
  Product11/1 -> Product11_pd1/1
  In2/1 -> Product11/2
  In1/1 -> Product11/1

== system gm_uz_pmsm_model_6LUT_pd_vnl/uz_pmsm_model_6LUT/Product110 ==
  In1 : Inport
  In2 : Inport  Port=2
  Product110 : Product  Inputs=**  OutDataTypeStr=double  SampleTime=1e-08
  Product110_pd1 : Delay  DelayLength=6
  Out1 : Outport
  wires:
  Product110_pd1/1 -> Out1/1
  Product110/1 -> Product110_pd1/1
  In2/1 -> Product110/2
  In1/1 -> Product110/1

== system gm_uz_pmsm_model_6LUT_pd_vnl/uz_pmsm_model_6LUT/Product111 ==
  In1 : Inport
  In2 : Inport  Port=2
  Product111 : Product  Inputs=**  OutDataTypeStr=double  SampleTime=1e-08
  Product111_pd1 : Delay  DelayLength=6
  Out1 : Outport
  wires:
  Product111_pd1/1 -> Out1/1
  Product111/1 -> Product111_pd1/1
  In2/1 -> Product111/2
  In1/1 -> Product111/1

== system gm_uz_pmsm_model_6LUT_pd_vnl/uz_pmsm_model_6LUT/Product112 ==
  In1 : Inport
  In2 : Inport  Port=2
  Product112 : Product  Inputs=**  OutDataTypeStr=double  SampleTime=1e-08
  Product112_pd1 : Delay  DelayLength=6
  Out1 : Outport
  wires:
  Product112_pd1/1 -> Out1/1
  Product112/1 -> Product112_pd1/1
  In2/1 -> Product112/2
  In1/1 -> Product112/1

== system gm_uz_pmsm_model_6LUT_pd_vnl/uz_pmsm_model_6LUT/Product113 ==
  In1 : Inport
  In2 : Inport  Port=2
  Product113 : Product  Inputs=*/  OutDataTypeStr=double  SampleTime=1e-08
  Product113_pd1 : Delay  DelayLength=31
  Out1 : Outport
  wires:
  Product113_pd1/1 -> Out1/1
  Product113/1 -> Product113_pd1/1
  In2/1 -> Product113/2
  In1/1 -> Product113/1

== system gm_uz_pmsm_model_6LUT_pd_vnl/uz_pmsm_model_6LUT/Product12 ==
  In1 : Inport
  In2 : Inport  Port=2
  Product12 : Product  Inputs=**  OutDataTypeStr=double  SampleTime=1e-08
  Product12_pd1 : Delay  DelayLength=6
  Out1 : Outport
  wires:
  Product12_pd1/1 -> Out1/1
  Product12/1 -> Product12_pd1/1
  In2/1 -> Product12/2
  In1/1 -> Product12/1

== system gm_uz_pmsm_model_6LUT_pd_vnl/uz_pmsm_model_6LUT/Product121 ==
  In1 : Inport
  In2 : Inport  Port=2
  Product121 : Product  Inputs=**  OutDataTypeStr=double  SampleTime=1e-08
  Product121_pd1 : Delay  DelayLength=6
  Out1 : Outport
  wires:
  Product121_pd1/1 -> Out1/1
  Product121/1 -> Product121_pd1/1
  In2/1 -> Product121/2
  In1/1 -> Product121/1

== system gm_uz_pmsm_model_6LUT_pd_vnl/uz_pmsm_model_6LUT/Product122 ==
  In1 : Inport
  In2 : Inport  Port=2
  Product122 : Product  Inputs=**  OutDataTypeStr=double  SampleTime=1e-08
  Product122_pd1 : Delay  DelayLength=6
  Out1 : Outport
  wires:
  Product122_pd1/1 -> Out1/1
  Product122/1 -> Product122_pd1/1
  In2/1 -> Product122/2
  In1/1 -> Product122/1

== system gm_uz_pmsm_model_6LUT_pd_vnl/uz_pmsm_model_6LUT/Product13 ==
  In1 : Inport
  In2 : Inport  Port=2
  Product13 : Product  Inputs=**  OutDataTypeStr=double  SampleTime=1e-08
  Product13_pd1 : Delay  DelayLength=6
  Out1 : Outport
  wires:
  Product13_pd1/1 -> Out1/1
  Product13/1 -> Product13_pd1/1
  In2/1 -> Product13/2
  In1/1 -> Product13/1

== system gm_uz_pmsm_model_6LUT_pd_vnl/uz_pmsm_model_6LUT/Product131 ==
  In1 : Inport
  In2 : Inport  Port=2
  Product131 : Product  Inputs=**  OutDataTypeStr=double  SampleTime=1e-08
  Product131_pd1 : Delay  DelayLength=6
  Out1 : Outport
  wires:
  Product131_pd1/1 -> Out1/1
  Product131/1 -> Product131_pd1/1
  In2/1 -> Product131/2
  In1/1 -> Product131/1

== system gm_uz_pmsm_model_6LUT_pd_vnl/uz_pmsm_model_6LUT/Product132 ==
  In1 : Inport
  In2 : Inport  Port=2
  Product132 : Product  Inputs=*/  OutDataTypeStr=double  SampleTime=1e-08
  Product132_pd1 : Delay  DelayLength=31
  Out1 : Outport
  wires:
  Product132_pd1/1 -> Out1/1
  Product132/1 -> Product132_pd1/1
  In2/1 -> Product132/2
  In1/1 -> Product132/1

== system gm_uz_pmsm_model_6LUT_pd_vnl/uz_pmsm_model_6LUT/Product133 ==
  In1 : Inport
  In2 : Inport  Port=2
  Product133 : Product  Inputs=*/  OutDataTypeStr=double  SampleTime=1e-08
  Product133_pd1 : Delay  DelayLength=31
  Out1 : Outport
  wires:
  Product133_pd1/1 -> Out1/1
  Product133/1 -> Product133_pd1/1
  In2/1 -> Product133/2
  In1/1 -> Product133/1

== system gm_uz_pmsm_model_6LUT_pd_vnl/uz_pmsm_model_6LUT/Product14 ==
  In1 : Inport
  In2 : Inport  Port=2
  Product14 : Product  Inputs=**  OutDataTypeStr=single  SampleTime=1e-08
  Product14_pd1 : Delay  DelayLength=6
  Out1 : Outport
  wires:
  Product14_pd1/1 -> Out1/1
  Product14/1 -> Product14_pd1/1
  In2/1 -> Product14/2
  In1/1 -> Product14/1

== system gm_uz_pmsm_model_6LUT_pd_vnl/uz_pmsm_model_6LUT/Product141 ==
  In1 : Inport
  In2 : Inport  Port=2
  Product141 : Product  Inputs=**  OutDataTypeStr=single  SampleTime=1e-08
  Product141_pd1 : Delay  DelayLength=6
  Out1 : Outport
  wires:
  Product141_pd1/1 -> Out1/1
  Product141/1 -> Product141_pd1/1
  In2/1 -> Product141/2
  In1/1 -> Product141/1

== system gm_uz_pmsm_model_6LUT_pd_vnl/uz_pmsm_model_6LUT/Product15 ==
  In1 : Inport
  In2 : Inport  Port=2
  Product15 : Product  Inputs=**  OutDataTypeStr=single  SampleTime=1e-08
  Product15_pd1 : Delay  DelayLength=6
  Out1 : Outport
  wires:
  Product15_pd1/1 -> Out1/1
  Product15/1 -> Product15_pd1/1
  In2/1 -> Product15/2
  In1/1 -> Product15/1

== system gm_uz_pmsm_model_6LUT_pd_vnl/uz_pmsm_model_6LUT/Product151 ==
  In1 : Inport
  In2 : Inport  Port=2
  Product151 : Product  Inputs=**  OutDataTypeStr=single  SampleTime=1e-08
  Product151_pd1 : Delay  DelayLength=6
  Out1 : Outport
  wires:
  Product151_pd1/1 -> Out1/1
  Product151/1 -> Product151_pd1/1
  In2/1 -> Product151/2
  In1/1 -> Product151/1

== system gm_uz_pmsm_model_6LUT_pd_vnl/uz_pmsm_model_6LUT/Product16 ==
  In1 : Inport
  In2 : Inport  Port=2
  Product16 : Product  Inputs=**  OutDataTypeStr=double  SampleTime=1e-08
  Product16_pd1 : Delay  DelayLength=6
  Out1 : Outport
  wires:
  Product16_pd1/1 -> Out1/1
  Product16/1 -> Product16_pd1/1
  In2/1 -> Product16/2
  In1/1 -> Product16/1

== system gm_uz_pmsm_model_6LUT_pd_vnl/uz_pmsm_model_6LUT/Product161 ==
  In1 : Inport
  In2 : Inport  Port=2
  Product161 : Product  Inputs=*/  OutDataTypeStr=double  SampleTime=1e-08
  Product161_pd1 : Delay  DelayLength=31
  Out1 : Outport
  wires:
  Product161_pd1/1 -> Out1/1
  Product161/1 -> Product161_pd1/1
  In2/1 -> Product161/2
  In1/1 -> Product161/1

== system gm_uz_pmsm_model_6LUT_pd_vnl/uz_pmsm_model_6LUT/Product162 ==
  In1 : Inport
  In2 : Inport  Port=2
  Product162 : Product  Inputs=*/  OutDataTypeStr=double  SampleTime=1e-08
  Product162_pd1 : Delay  DelayLength=31
  Out1 : Outport
  wires:
  Product162_pd1/1 -> Out1/1
  Product162/1 -> Product162_pd1/1
  In2/1 -> Product162/2
  In1/1 -> Product162/1

== system gm_uz_pmsm_model_6LUT_pd_vnl/uz_pmsm_model_6LUT/Product17 ==
  In1 : Inport
  In2 : Inport  Port=2
  Product17 : Product  Inputs=**  OutDataTypeStr=double  SampleTime=1e-08
  Product17_pd1 : Delay  DelayLength=6
  Out1 : Outport
  wires:
  Product17_pd1/1 -> Out1/1
  Product17/1 -> Product17_pd1/1
  In2/1 -> Product17/2
  In1/1 -> Product17/1

== system gm_uz_pmsm_model_6LUT_pd_vnl/uz_pmsm_model_6LUT/Product18 ==
  In1 : Inport
  In2 : Inport  Port=2
  Product18 : Product  Inputs=**  OutDataTypeStr=double  SampleTime=1e-08
  Product18_pd1 : Delay  DelayLength=6
  Out1 : Outport
  wires:
  Product18_pd1/1 -> Out1/1
  Product18/1 -> Product18_pd1/1
  In2/1 -> Product18/2
  In1/1 -> Product18/1

== system gm_uz_pmsm_model_6LUT_pd_vnl/uz_pmsm_model_6LUT/Product19 ==
  In1 : Inport
  In2 : Inport  Port=2
  Product19 : Product  Inputs=**  OutDataTypeStr=double  SampleTime=1e-08
  Product19_pd1 : Delay  DelayLength=6
  Out1 : Outport
  wires:
  Product19_pd1/1 -> Out1/1
  Product19/1 -> Product19_pd1/1
  In2/1 -> Product19/2
  In1/1 -> Product19/1

== system gm_uz_pmsm_model_6LUT_pd_vnl/uz_pmsm_model_6LUT/Product2 ==
  In1 : Inport
  In2 : Inport  Port=2
  Product2 : Product  Inputs=**  OutDataTypeStr=double  SampleTime=1e-08
  Product2_pd1 : Delay  DelayLength=6
  Out1 : Outport
  wires:
  Product2_pd1/1 -> Out1/1
  Product2/1 -> Product2_pd1/1
  In2/1 -> Product2/2
  In1/1 -> Product2/1

== system gm_uz_pmsm_model_6LUT_pd_vnl/uz_pmsm_model_6LUT/Product20 ==
  In1 : Inport
  In2 : Inport  Port=2
  Product20 : Product  Inputs=**  OutDataTypeStr=double  SampleTime=1e-08
  Product20_pd1 : Delay  DelayLength=6
  Out1 : Outport
  wires:
  Product20_pd1/1 -> Out1/1
  Product20/1 -> Product20_pd1/1
  In2/1 -> Product20/2
  In1/1 -> Product20/1

== system gm_uz_pmsm_model_6LUT_pd_vnl/uz_pmsm_model_6LUT/Product201 ==
  In1 : Inport
  In2 : Inport  Port=2
  Product201 : Product  Inputs=**  OutDataTypeStr=double  SampleTime=1e-08
  Product201_pd1 : Delay  DelayLength=6
  Out1 : Outport
  wires:
  Product201_pd1/1 -> Out1/1
  Product201/1 -> Product201_pd1/1
  In2/1 -> Product201/2
  In1/1 -> Product201/1

== system gm_uz_pmsm_model_6LUT_pd_vnl/uz_pmsm_model_6LUT/Product202 ==
  In1 : Inport
  In2 : Inport  Port=2
  Product202 : Product  Inputs=**  OutDataTypeStr=double  SampleTime=1e-08
  Product202_pd1 : Delay  DelayLength=6
  Out1 : Outport
  wires:
  Product202_pd1/1 -> Out1/1
  Product202/1 -> Product202_pd1/1
  In2/1 -> Product202/2
  In1/1 -> Product202/1

== system gm_uz_pmsm_model_6LUT_pd_vnl/uz_pmsm_model_6LUT/Product203 ==
  In1 : Inport
  In2 : Inport  Port=2
  Product203 : Product  Inputs=**  OutDataTypeStr=double  SampleTime=1e-08
  Product203_pd1 : Delay  DelayLength=6
  Out1 : Outport
  wires:
  Product203_pd1/1 -> Out1/1
  Product203/1 -> Product203_pd1/1
  In2/1 -> Product203/2
  In1/1 -> Product203/1

== system gm_uz_pmsm_model_6LUT_pd_vnl/uz_pmsm_model_6LUT/Product204 ==
  In1 : Inport
  In2 : Inport  Port=2
  Product204 : Product  Inputs=**  OutDataTypeStr=double  SampleTime=1e-08
  Product204_pd1 : Delay  DelayLength=6
  Out1 : Outport
  wires:
  Product204_pd1/1 -> Out1/1
  Product204/1 -> Product204_pd1/1
  In2/1 -> Product204/2
  In1/1 -> Product204/1

== system gm_uz_pmsm_model_6LUT_pd_vnl/uz_pmsm_model_6LUT/Product205 ==
  In1 : Inport
  In2 : Inport  Port=2
  Product205 : Product  Inputs=**  OutDataTypeStr=double  SampleTime=1e-08
  Product205_pd1 : Delay  DelayLength=6
  Out1 : Outport
  wires:
  Product205_pd1/1 -> Out1/1
  Product205/1 -> Product205_pd1/1
  In2/1 -> Product205/2
  In1/1 -> Product205/1

== system gm_uz_pmsm_model_6LUT_pd_vnl/uz_pmsm_model_6LUT/Product206 ==
  In1 : Inport
  In2 : Inport  Port=2
  Product206 : Product  Inputs=**  OutDataTypeStr=double  SampleTime=1e-08
  Product206_pd1 : Delay  DelayLength=6
  Out1 : Outport
  wires:
  Product206_pd1/1 -> Out1/1
  Product206/1 -> Product206_pd1/1
  In2/1 -> Product206/2
  In1/1 -> Product206/1

== system gm_uz_pmsm_model_6LUT_pd_vnl/uz_pmsm_model_6LUT/Product207 ==
  In1 : Inport
  In2 : Inport  Port=2
  Product207 : Product  Inputs=**  OutDataTypeStr=double  SampleTime=1e-08
  Product207_pd1 : Delay  DelayLength=6
  Out1 : Outport
  wires:
  Product207_pd1/1 -> Out1/1
  Product207/1 -> Product207_pd1/1
  In2/1 -> Product207/2
  In1/1 -> Product207/1

== system gm_uz_pmsm_model_6LUT_pd_vnl/uz_pmsm_model_6LUT/Product21 ==
  In1 : Inport
  In2 : Inport  Port=2
  Product21 : Product  Inputs=**  OutDataTypeStr=double  SampleTime=1e-08
  Product21_pd1 : Delay  DelayLength=6
  Out1 : Outport
  wires:
  Product21_pd1/1 -> Out1/1
  Product21/1 -> Product21_pd1/1
  In2/1 -> Product21/2
  In1/1 -> Product21/1

== system gm_uz_pmsm_model_6LUT_pd_vnl/uz_pmsm_model_6LUT/Product211 ==
  In1 : Inport
  In2 : Inport  Port=2
  Product211 : Product  Inputs=*/  OutDataTypeStr=double  SampleTime=1e-08
  Product211_pd1 : Delay  DelayLength=31
  Out1 : Outport
  wires:
  Product211_pd1/1 -> Out1/1
  Product211/1 -> Product211_pd1/1
  In2/1 -> Product211/2
  In1/1 -> Product211/1

== system gm_uz_pmsm_model_6LUT_pd_vnl/uz_pmsm_model_6LUT/Product22 ==
  In1 : Inport
  In2 : Inport  Port=2
  Product22 : Product  Inputs=**  OutDataTypeStr=double  SampleTime=1e-08
  Product22_pd1 : Delay  DelayLength=6
  Out1 : Outport
  wires:
  Product22_pd1/1 -> Out1/1
  Product22/1 -> Product22_pd1/1
  In2/1 -> Product22/2
  In1/1 -> Product22/1

== system gm_uz_pmsm_model_6LUT_pd_vnl/uz_pmsm_model_6LUT/Product23 ==
  In1 : Inport
  In2 : Inport  Port=2
  Product23 : Product  Inputs=**  OutDataTypeStr=double  SampleTime=1e-08
  Product23_pd1 : Delay  DelayLength=6
  Out1 : Outport
  wires:
  Product23_pd1/1 -> Out1/1
  Product23/1 -> Product23_pd1/1
  In2/1 -> Product23/2
  In1/1 -> Product23/1

== system gm_uz_pmsm_model_6LUT_pd_vnl/uz_pmsm_model_6LUT/Product24 ==
  In1 : Inport
  In2 : Inport  Port=2
  Product24 : Product  Inputs=**  OutDataTypeStr=double  SampleTime=1e-08
  Product24_pd1 : Delay  DelayLength=6
  Out1 : Outport
  wires:
  Product24_pd1/1 -> Out1/1
  Product24/1 -> Product24_pd1/1
  In2/1 -> Product24/2
  In1/1 -> Product24/1

== system gm_uz_pmsm_model_6LUT_pd_vnl/uz_pmsm_model_6LUT/Product25 ==
  In1 : Inport
  In2 : Inport  Port=2
  Product25 : Product  Inputs=**  OutDataTypeStr=double  SampleTime=1e-08
  Product25_pd1 : Delay  DelayLength=6
  Out1 : Outport
  wires:
  Product25_pd1/1 -> Out1/1
  Product25/1 -> Product25_pd1/1
  In2/1 -> Product25/2
  In1/1 -> Product25/1

== system gm_uz_pmsm_model_6LUT_pd_vnl/uz_pmsm_model_6LUT/Product3 ==
  In1 : Inport
  In2 : Inport  Port=2
  Product3 : Product  Inputs=**  OutDataTypeStr=double  SampleTime=1e-08
  Product3_pd1 : Delay  DelayLength=6
  Out1 : Outport
  wires:
  Product3_pd1/1 -> Out1/1
  Product3/1 -> Product3_pd1/1
  In2/1 -> Product3/2
  In1/1 -> Product3/1

== system gm_uz_pmsm_model_6LUT_pd_vnl/uz_pmsm_model_6LUT/Product31 ==
  In1 : Inport
  In2 : Inport  Port=2
  Product31 : Product  Inputs=**  OutDataTypeStr=double  SampleTime=1e-08
  Product31_pd1 : Delay  DelayLength=6
  Out1 : Outport
  wires:
  Product31_pd1/1 -> Out1/1
  Product31/1 -> Product31_pd1/1
  In2/1 -> Product31/2
  In1/1 -> Product31/1

== system gm_uz_pmsm_model_6LUT_pd_vnl/uz_pmsm_model_6LUT/Product32 ==
  In1 : Inport
  In2 : Inport  Port=2
  Product32 : Product  Inputs=**  OutDataTypeStr=double  SampleTime=1e-08
  Product32_pd1 : Delay  DelayLength=6
  Out1 : Outport
  wires:
  Product32_pd1/1 -> Out1/1
  Product32/1 -> Product32_pd1/1
  In2/1 -> Product32/2
  In1/1 -> Product32/1

== system gm_uz_pmsm_model_6LUT_pd_vnl/uz_pmsm_model_6LUT/Product33 ==
  In1 : Inport
  In2 : Inport  Port=2
  Product33 : Product  Inputs=**  OutDataTypeStr=double  SampleTime=1e-08
  Product33_pd1 : Delay  DelayLength=6
  Out1 : Outport
  wires:
  Product33_pd1/1 -> Out1/1
  Product33/1 -> Product33_pd1/1
  In2/1 -> Product33/2
  In1/1 -> Product33/1

== system gm_uz_pmsm_model_6LUT_pd_vnl/uz_pmsm_model_6LUT/Product34 ==
  In1 : Inport
  In2 : Inport  Port=2
  Product34 : Product  Inputs=**  OutDataTypeStr=double  SampleTime=1e-08
  Product34_pd1 : Delay  DelayLength=6
  Out1 : Outport
  wires:
  Product34_pd1/1 -> Out1/1
  Product34/1 -> Product34_pd1/1
  In2/1 -> Product34/2
  In1/1 -> Product34/1

== system gm_uz_pmsm_model_6LUT_pd_vnl/uz_pmsm_model_6LUT/Product35 ==
  In1 : Inport
  In2 : Inport  Port=2
  Product35 : Product  Inputs=**  OutDataTypeStr=double  SampleTime=1e-08
  Product35_pd1 : Delay  DelayLength=6
  Out1 : Outport
  wires:
  Product35_pd1/1 -> Out1/1
  Product35/1 -> Product35_pd1/1
  In2/1 -> Product35/2
  In1/1 -> Product35/1

== system gm_uz_pmsm_model_6LUT_pd_vnl/uz_pmsm_model_6LUT/Product36 ==
  In1 : Inport
  In2 : Inport  Port=2
  Product36 : Product  Inputs=**  OutDataTypeStr=double  SampleTime=1e-08
  Product36_pd1 : Delay  DelayLength=6
  Out1 : Outport
  wires:
  Product36_pd1/1 -> Out1/1
  Product36/1 -> Product36_pd1/1
  In2/1 -> Product36/2
  In1/1 -> Product36/1

== system gm_uz_pmsm_model_6LUT_pd_vnl/uz_pmsm_model_6LUT/Product37 ==
  In1 : Inport
  In2 : Inport  Port=2
  Product37 : Product  Inputs=**  OutDataTypeStr=double  SampleTime=1e-08
  Product37_pd1 : Delay  DelayLength=6
  Out1 : Outport
  wires:
  Product37_pd1/1 -> Out1/1
  Product37/1 -> Product37_pd1/1
  In2/1 -> Product37/2
  In1/1 -> Product37/1

== system gm_uz_pmsm_model_6LUT_pd_vnl/uz_pmsm_model_6LUT/Product4 ==
  In1 : Inport
  In2 : Inport  Port=2
  Product4 : Product  Inputs=**  OutDataTypeStr=double  SampleTime=1e-08
  Product4_pd1 : Delay  DelayLength=6
  Out1 : Outport
  wires:
  Product4_pd1/1 -> Out1/1
  Product4/1 -> Product4_pd1/1
  In2/1 -> Product4/2
  In1/1 -> Product4/1
